simulink model "Test2_1"  (R2021a)
(part 2 of 2)

  Line 89 : spsDistributedParametersLineLib/Distributed Parameters Line  Phases=3  Length=0.02  Frequency=50  Resistance=[0.646656091154803 0.0486237908083191 0.0486712220507153;0.0486237908083191 0.646561225344642 0.0486237934466192;0.0486712220507153 0.0486237934466192 0.646656091154803]  Inductance=[0.00282448912315926 0.00133270803418135 0.00132951476746136;0.00133270803418135 0.00282479813276775 0.00133799988507366;0.00132951476746136 0.00133799988507366 0.00282448912315926]  Capacitance=[7.89543174552926e-09 -1.85986777702161e-09 -1.7901190036642e-09;-1.85986777702161e-09 7.82540023894543e-09 -1.8957321828871e-09;-1.7901190036642e-09 -1.8957321828871e-09 7.91264394645417e-09]  x1=[153.230370640917 2391.26534326387 2395.45779665592;314.159265358979 314.159265358979 314.159265358979;0.9381426054202 -0.865117419435394 -2.43426019857906]  x2=[153.230402844459 2391.26073889825 2395.45319480697;314.159265358979 314.159265358979 314.159265358979;0.93814254539382 -0.865117633756149 -2.43426040689413]  x3=[0.134091150426205 5.82873242831537 5.88568625716513;314.159265358979 314.159265358979 314.159265358979;0.931522107244716 -0.837575635614275 -2.40695052925784]  x4=[0.133861464896509 6.3462381763928 6.40423326646663;314.159265358979 314.159265358979 314.159265358979;0.944744271874414 -0.890435947392576 -2.45938130511451]  x5=9.5829454252223e-08  V1=ones(3,3)  V2=ones(3,3)  I1=ones(3,3)  I2=ones(3,3)  nHarmo=1  Measurements=None  Decoupling=off  VsMag0=0  VrMag0=0  VsAngle0=0  VrAngle0=0  IsMag0=0  IrMag0=0  IsAngle0=0  IrAngle0=0
      settings: SourceProductBaseCode=PS
  Line 9 : spsDistributedParametersLineLib/Distributed Parameters Line  Phases=3  Length=0.02  Frequency=50  Resistance=[0.646656091154803 0.0486237908083191 0.0486712220507153;0.0486237908083191 0.646561225344642 0.0486237934466192;0.0486712220507153 0.0486237934466192 0.646656091154803]  Inductance=[0.00282448912315926 0.00133270803418135 0.00132951476746136;0.00133270803418135 0.00282479813276775 0.00133799988507366;0.00132951476746136 0.00133799988507366 0.00282448912315926]  Capacitance=[7.89543174552926e-09 -1.85986777702161e-09 -1.7901190036642e-09;-1.85986777702161e-09 7.82540023894543e-09 -1.8957321828871e-09;-1.7901190036642e-09 -1.8957321828871e-09 7.91264394645417e-09]  x1=[139.613784628439 4217.52722308047 4217.62642474081;314.159265358979 314.159265358979 314.159265358979;0.931225166408948 1.89080004922946 -2.8202976922573]  x2=[139.613822815392 4217.52006491205 4217.61927834542;314.159265358979 314.159265358979 314.159265358979;0.931225429888519 1.89079965963336 -2.82029807495107]  x3=[0.123373305824632 10.2981496913263 10.380801790438;314.159265358979 314.159265358979 314.159265358979;0.926779421621701 1.91078292702978 -2.8004554345958]  x4=[0.120765224807825 11.1715858882522 11.2542853331702;314.159265358979 314.159265358979 314.159265358979;0.935736759138729 1.87235633522372 -2.83862312372742]  x5=9.5829454252223e-08  V1=ones(3,3)  V2=ones(3,3)  I1=ones(3,3)  I2=ones(3,3)  nHarmo=1  Measurements=None  Decoupling=off  VsMag0=0  VrMag0=0  VsAngle0=0  VrAngle0=0  IsMag0=0  IrMag0=0  IsAngle0=0  IrAngle0=0
      settings: SourceProductBaseCode=PS
  Line im1 : spsDistributedParametersLineLib/Distributed Parameters Line  Phases=3  Length=1e-10  Frequency=50  Resistance=[0.646656091154803 0.0486237908083191 0.0486712220507153;0.0486237908083191 0.646561225344642 0.0486237934466192;0.0486712220507153 0.0486237934466192 0.646656091154803]  Inductance=[0.00282448912315926 0.00133270803418135 0.00132951476746136;0.00133270803418135 0.00282479813276775 0.00133799988507366;0.00132951476746136 0.00133799988507366 0.00282448912315926]  Capacitance=[7.89543174552926e-09 -1.85986777702161e-09 -1.7901190036642e-09;-1.85986777702161e-09 7.82540023894543e-09 -1.8957321828871e-09;-1.7901190036642e-09 -1.8957321828871e-09 7.91264394645417e-09]  x1=[139.600491467614 4218.81584590389 4218.91451607394;314.159265358979 314.159265358979 314.159265358979;0.93120240765686 1.89102757934652 -2.82007159456862]  x2=[139.600491467484 4218.81584590393 4218.91451607418;314.159265358979 314.159265358979 314.159265358979;0.931202407653615 1.89102757934648 -2.82007159456862]  x3=[2.39495104418877 10.0531520558199 13.4523376279678;314.159265358979 314.159265358979 314.159265358979;-2.07306138977406 1.7159728748214 -2.96321720619588]  x4=[2.63858020709018 11.6972228256435 8.53725478011855;314.159265358979 314.159265358979 314.159265358979;1.05327657505423 2.04091940379862 -2.59297720135789]  x5=4.79147271261115e-16  V1=ones(3,3)  V2=ones(3,3)  I1=ones(3,3)  I2=ones(3,3)  nHarmo=1  Measurements=None  Decoupling=off  VsMag0=0  VrMag0=0  VsAngle0=0  VrAngle0=0  IsMag0=0  IrMag0=0  IsAngle0=0  IrAngle0=0
      settings: SourceProductBaseCode=PS
  Line im2 : spsDistributedParametersLineLib/Distributed Parameters Line  Phases=3  Length=1e-10  Frequency=50  Resistance=[0.646656091154803 0.0486237908083191 0.0486712220507153;0.0486237908083191 0.646561225344642 0.0486237934466192;0.0486712220507153 0.0486237934466192 0.646656091154803]  Inductance=[0.00282448912315926 0.00133270803418135 0.00132951476746136;0.00133270803418135 0.00282479813276775 0.00133799988507366;0.00132951476746136 0.00133799988507366 0.00282448912315926]  Capacitance=[7.89543174552926e-09 -1.85986777702161e-09 -1.7901190036642e-09;-1.85986777702161e-09 7.82540023894543e-09 -1.8957321828871e-09;-1.7901190036642e-09 -1.8957321828871e-09 7.91264394645417e-09]  x1=[153.212558124086 2392.15576627611 2396.34818431222;314.159265358979 314.159265358979 314.159265358979;0.938198757168088 -0.864957859131465 -2.4341019124231]  x2=[153.212558124091 2392.15576627603 2396.34818431214;314.159265358979 314.159265358979 314.159265358979;0.938198757168096 -0.864957859131481 -2.43410191242311]  x3=[0.150374507197116 4.9941389131791 5.06923933643373;314.159265358979 314.159265358979 314.159265358979;0.783798645997587 -0.817862247865617 -2.376387681184]  x4=[0.120456415579041 7.18402866882818 7.23580636001522;314.159265358979 314.159265358979 314.159265358979;1.11210397866224 -0.897495860417821 -2.47460068555332]  x5=4.79147271261115e-16  V1=ones(3,3)  V2=ones(3,3)  I1=ones(3,3)  I2=ones(3,3)  nHarmo=1  Measurements=None  Decoupling=off  VsMag0=0  VrMag0=0  VsAngle0=0  VrAngle0=0  IsMag0=0  IrMag0=0  IsAngle0=0  IrAngle0=0
      settings: SourceProductBaseCode=PS
  Line im3 : spsDistributedParametersLineLib/Distributed Parameters Line  Phases=3  Length=1e-10  Frequency=50  Resistance=[0.646656091154803 0.0486237908083191 0.0486712220507153;0.0486237908083191 0.646561225344642 0.0486237934466192;0.0486712220507153 0.0486237934466192 0.646656091154803]  Inductance=[0.00282448912315926 0.00133270803418135 0.00132951476746136;0.00133270803418135 0.00282479813276775 0.00133799988507366;0.00132951476746136 0.00133799988507366 0.00282448912315926]  Capacitance=[7.89543174552926e-09 -1.85986777702161e-09 -1.7901190036642e-09;-1.85986777702161e-09 7.82540023894543e-09 -1.8957321828871e-09;-1.7901190036642e-09 -1.8957321828871e-09 7.91264394645417e-09]  x1=[138.811982406861 4221.87237170443 4226.20282418839;314.159265358979 314.159265358979 314.159265358979;0.909247916230907 -0.556815898274562 -2.12771519143661]  x2=[138.811982407814 4221.8723715327 4226.20282401679;314.159265358979 314.159265358979 314.159265358979;0.909247916234134 -0.556815898289708 -2.12771519145178]  x3=[5.7114352671611 2399.57047495897 2405.23950831528;314.159265358979 314.159265358979 314.159265358979;0.198532164333906 2.27374576995704 0.707186662876006]  x4=[5.52541559624089 2420.03219700396 2425.91155689626;314.159265358979 314.159265358979 314.159265358979;-2.97166603107008 -0.865128065419886 -2.43170878274322]  x5=4.79147271261115e-16  V1=ones(3,3)  V2=ones(3,3)  I1=ones(3,3)  I2=ones(3,3)  nHarmo=1  Measurements=None  Decoupling=off  VsMag0=0  VrMag0=0  VsAngle0=0  VrAngle0=0  IsMag0=0  IrMag0=0  IsAngle0=0  IrAngle0=0
      settings: SourceProductBaseCode=PS
  Load {1..2,11,13,8041,8173} (6 alike) : spsThreePhaseSeriesRLCLoadLib/Three-Phase Series RLC Load  LConnTagsString=A|B|C  Configuration=Delta  NominalVoltage=11000  Vabc=[1e3 1e3 1e3]  Vabcp=[1e3 1e3 1e3]  NominalFrequency=50  UnbalancedPower=off  ActivePower=28052.64  InductivePower=13586.514  CapacitivePower=0  Pabc=[10e3 9e3 11e3]  QLabc=[100 90 110]  QCabc=[100 90 110]  Pabcp=[10e3 9e3 11e3]  QLabcp=[100 90 110]  QCabcp=[100 90 110]  Measurements=None  LoadType=constant Z
  Load 10 : spsThreePhaseSeriesRLCLoadLib/Three-Phase Series RLC Load  LConnTagsString=A|B|C  Configuration=Delta  NominalVoltage=11000  Vabc=[1e3 1e3 1e3]  Vabcp=[1e3 1e3 1e3]  NominalFrequency=50  UnbalancedPower=off  ActivePower=17532.9  InductivePower=8491.571  CapacitivePower=0  Pabc=[10e3 9e3 11e3]  QLabc=[100 90 110]  QCabc=[100 90 110]  Pabcp=[10e3 9e3 11e3]  QLabcp=[100 90 110]  QCabcp=[100 90 110]  Measurements=None  LoadType=constant Z
  Load 12 : spsThreePhaseSeriesRLCLoadLib/Three-Phase Series RLC Load  LConnTagsString=A|B|C  Configuration=Delta  NominalVoltage=11000  Vabc=[1e3 1e3 1e3]  Vabcp=[1e3 1e3 1e3]  NominalFrequency=50  UnbalancedPower=off  ActivePower=17532.9  InductivePower=8491.571  CapacitivePower=0  Pabc=[10e3 9e3 11e3]  QLabc=[100 90 110]  QCabc=[100 90 110]  Pabcp=[10e3 9e3 11e3]  QLabcp=[100 90 110]  QCabcp=[100 90 110]  Measurements=None  LoadType=constant Z
  Load {3,6,14,17,8287,8485} (6 alike) : spsThreePhaseSeriesRLCLoadLib/Three-Phase Series RLC Load  LConnTagsString=A|B|C  Configuration=Delta  NominalVoltage=11000  Vabc=[1e3 1e3 1e3]  Vabcp=[1e3 1e3 1e3]  NominalFrequency=50  UnbalancedPower=off  ActivePower=35065.8  InductivePower=16983.142  CapacitivePower=0  Pabc=[10e3 9e3 11e3]  QLabc=[100 90 110]  QCabc=[100 90 110]  Pabcp=[10e3 9e3 11e3]  QLabcp=[100 90 110]  QCabcp=[100 90 110]  Measurements=None  LoadType=constant Z
  Load {4,9,15,20,8293,8733} (6 alike) : spsThreePhaseSeriesRLCLoadLib/Three-Phase Series RLC Load  LConnTagsString=A|B|C  Configuration=Delta  NominalVoltage=11000  Vabc=[1e3 1e3 1e3]  Vabcp=[1e3 1e3 1e3]  NominalFrequency=50  UnbalancedPower=off  ActivePower=7013.16  InductivePower=3396.628  CapacitivePower=0  Pabc=[10e3 9e3 11e3]  QLabc=[100 90 110]  QCabc=[100 90 110]  Pabcp=[10e3 9e3 11e3]  QLabcp=[100 90 110]  QCabcp=[100 90 110]  Measurements=None  LoadType=constant Z
  Load {5,7,16,18,8424,8551} (6 alike) : spsThreePhaseSeriesRLCLoadLib/Three-Phase Series RLC Load  LConnTagsString=A|B|C  Configuration=Delta  NominalVoltage=11000  Vabc=[1e3 1e3 1e3]  Vabcp=[1e3 1e3 1e3]  NominalFrequency=50  UnbalancedPower=off  ActivePower=11221.056  InductivePower=5434.605  CapacitivePower=0  Pabc=[10e3 9e3 11e3]  QLabc=[100 90 110]  QCabc=[100 90 110]  Pabcp=[10e3 9e3 11e3]  QLabcp=[100 90 110]  QCabcp=[100 90 110]  Measurements=None  LoadType=constant Z
  Load 19 : spsThreePhaseSeriesRLCLoadLib/Three-Phase Series RLC Load  LConnTagsString=A|B|C  Configuration=Delta  NominalVoltage=11000  Vabc=[1e3 1e3 1e3]  Vabcp=[1e3 1e3 1e3]  NominalFrequency=50  UnbalancedPower=off  ActivePower=280.526  InductivePower=135.865  CapacitivePower=0  Pabc=[10e3 9e3 11e3]  QLabc=[100 90 110]  QCabc=[100 90 110]  Pabcp=[10e3 9e3 11e3]  QLabcp=[100 90 110]  QCabcp=[100 90 110]  Measurements=None  LoadType=constant Z
  Load 8 : spsThreePhaseSeriesRLCLoadLib/Three-Phase Series RLC Load  LConnTagsString=A|B|C  Configuration=Delta  NominalVoltage=11000  Vabc=[1e3 1e3 1e3]  Vabcp=[1e3 1e3 1e3]  NominalFrequency=50  UnbalancedPower=off  ActivePower=280.526  InductivePower=135.865  CapacitivePower=0  Pabc=[10e3 9e3 11e3]  QLabc=[100 90 110]  QCabc=[100 90 110]  Pabcp=[10e3 9e3 11e3]  QLabcp=[100 90 110]  QCabcp=[100 90 110]  Measurements=None  LoadType=constant Z
  Load 8605 : spsThreePhaseSeriesRLCLoadLib/Three-Phase Series RLC Load  LConnTagsString=A|B|C  Configuration=Delta  NominalVoltage=11000  Vabc=[1e3 1e3 1e3]  Vabcp=[1e3 1e3 1e3]  NominalFrequency=50  UnbalancedPower=off  ActivePower=280.526  InductivePower=135.865  CapacitivePower=0  Pabc=[10e3 9e3 11e3]  QLabc=[100 90 110]  QCabc=[100 90 110]  Pabcp=[10e3 9e3 11e3]  QLabcp=[100 90 110]  QCabcp=[100 90 110]  Measurements=None  LoadType=constant Z
  Load 8737 : spsThreePhaseSeriesRLCLoadLib/Three-Phase Series RLC Load  LConnTagsString=A|B|C  Configuration=Delta  NominalVoltage=11000  Vabc=[1e3 1e3 1e3]  Vabcp=[1e3 1e3 1e3]  NominalFrequency=50  UnbalancedPower=off  ActivePower=17532.9  InductivePower=8491.571  CapacitivePower=0  Pabc=[10e3 9e3 11e3]  QLabc=[100 90 110]  QCabc=[100 90 110]  Pabcp=[10e3 9e3 11e3]  QLabcp=[100 90 110]  QCabcp=[100 90 110]  Measurements=None  LoadType=constant Z
  R{1..3,5} (4 alike) : spsThreePhaseVIMeasurementLib/Three-Phase V-I Measurement  VoltageMeasurement=phase-to-ground  SetLabelV=off  LabelV=Vabc  Vpu=off  VpuLL=off  CurrentMeasurement=yes  SetLabelI=off  LabelI=Iabc  Ipu=off  Pbase=100e6  Vbase=500e3  OutputType=Complex  PhasorSimulation=on  PSBequivalent=0
  Scope R{1..3,5} (4 alike) : Scope  NumInputPorts=2
  Source PC1_TT2 : spsThreePhaseSourceLib/Three-Phase Source  InternalConnection=Yn  VoltagePhases=off  Voltage=10000  PhaseAngle=0  Voltage_phases=[25e3 25e3 25e3]/sqrt(3)  PhaseAngles_phases=[0 -120 +120]  Frequency=50  NonIdealSource=on  SpecifyImpedance=off  Resistance=0.14  Inductance=0.0031831  ShortCircuitLevel=100e6  BaseVoltage=25e3  XRratio=7  BusType=swing  Pref=10e3  Qref=0  Prefabc=[10e3, 10e3, 10e3]  Qrefabc=[0, 0, 0]  Qmin=-inf  Qmax=inf
  Source Zn : spsSeriesRLCBranchLib/Series RLC Branch  LConnTagsString=__new0  RConnTagsString=__new0  BranchType=RL  Resistance=0.001  Inductance=3.1831e-06  SetiL0=off  InitialCurrent=0  Capacitance=0  Setx0=off  InitialVoltage=0  Measurements=None
  powergui : spspowerguiLib/powergui  Priority=1  SimulationMode=Phasor  SampleTime=50e-6  frequency=50  Iterations=50  frequencyindice=50  Pbase=100e6  ErrMax=1e-4  UnitsV=kV  UnitsW=MW  buscounter=0  FunctionMessages=off  echomessages=off  EnableUseOfTLC=off  CurrentSourceSwitches=off  DisableSnubberDevices=off  DisableRonSwitches=off  DisableVfSwitches=off  DisplayEquations=off  AutomaticDiscreteSolvers=off  SolverType=Tustin/Backward Euler (TBE)  Interpol=off  ExternalGateDelay=off  methode=off  Ts=10  x0status=blocks  SPID=off  SwTol=0  HookPort=off  NonlinearTolerance=1e-4  nMaxIteration=100  ContinueOnMaxIteration=off  RestoreLinks=warning  ResistiveCurrentMeasurement=off  Frange=[0:2:500]  Ylog=off  Xlog=on  ShowGrid=off  save=off  variable=ZData  structure=0  ZoomFFT=off  StartTime=0.0  cycles=1  DisplayStyle=1  fundamental=60  FreqAxis=off  MaxFrequency=1000  frequencyindicesteady=1  RmsSteady=1  display=off
  wires:
  R5/1 -> Scope R5/1
  R2/2 -> Scope R2/2
  R2/1 -> Scope R2/1
  R5/2 -> Scope R5/2
  R1/2 -> Scope R1/2
  R1/1 -> Scope R1/1
  R3/2 -> Scope R3/2
  R3/1 -> Scope R3/1
  connections:
  Source Zn/RConn1 -- Source PC1_TT2/LConn1
  Source Zn/LConn1 -- Ground/LConn1
  Line 58/LConn1 -- Line 57/LConn1 -- Line 56/RConn1
  Line 58/LConn2 -- Line 57/LConn2 -- Line 56/RConn2
  Line 58/LConn3 -- Line 57/LConn3 -- Line 56/RConn3
  Line 81/RConn1 -- Load 11/LConn1
  Line 81/RConn2 -- Load 11/LConn2
  Line 81/RConn3 -- Load 11/LConn3
  Load 20/LConn1 -- Line 42/RConn1
  Load 20/LConn2 -- Line 42/RConn2
  Load 20/LConn3 -- Line 42/RConn3
  Line 49/LConn1 -- Line 48/LConn1 -- Line 47/RConn1
  Line 49/LConn2 -- Line 48/LConn2 -- Line 47/RConn2
  Line 49/LConn3 -- Line 48/LConn3 -- Line 47/RConn3
  Line 28/RConn1 -- Load 1/LConn1
  Line 28/RConn2 -- Load 1/LConn2
  Line 28/RConn3 -- Load 1/LConn3
  Line 23/RConn1 -- Load 8/LConn1
  Line 23/RConn2 -- Load 8/LConn2
  Line 23/RConn3 -- Load 8/LConn3
  Line 74/LConn1 -- R2/RConn1
  Line 74/LConn2 -- R2/RConn2
  Line 74/LConn3 -- R2/RConn3
  Line 15/LConn1 -- Line 14/LConn1 -- Line 13/RConn1
  Line 15/LConn2 -- Line 14/LConn2 -- Line 13/RConn2
  Line 15/LConn3 -- Line 14/LConn3 -- Line 13/RConn3
  Line 17/LConn1 -- Line 16/LConn1 -- Line im1/RConn1
  Line 17/LConn2 -- Line 16/LConn2 -- Line im1/RConn2
  Line 16/LConn3 -- Line 17/LConn3 -- Line im1/RConn3
  Line 20/LConn1 -- Line 19/LConn1 -- Line 21/RConn1
  Line 20/LConn2 -- Line 19/LConn2 -- Line 21/RConn2
  Line 20/LConn3 -- Line 19/LConn3 -- Line 21/RConn3
  Load 13/LConn1 -- Line 83/LConn1 -- Line 87/RConn1 -- Line 41/LConn1
  Load 13/LConn2 -- Line 83/LConn2 -- Line 87/RConn2 -- Line 41/LConn2
  Line 41/LConn3 -- Load 13/LConn3 -- Line 87/RConn3 -- Line 83/LConn3
  Line im2/LConn1 -- R3/RConn1
  Line im2/LConn2 -- R3/RConn2
  Line im2/LConn3 -- R3/RConn3
  Line 19/RConn1 -- R1/LConn1
  Line 19/RConn2 -- R1/LConn2
  Line 19/RConn3 -- R1/LConn3
  Load 10/LConn1 -- Line 9/RConn1
  Load 10/LConn2 -- Line 9/RConn2
  Load 10/LConn3 -- Line 9/RConn3
  Source PC1_TT2/RConn1 -- R2/LConn1
  Source PC1_TT2/RConn2 -- R2/LConn2
  Source PC1_TT2/RConn3 -- R2/LConn3
  Line 71/LConn1 -- Line 70/LConn1 -- Line 72/RConn1
  Line 71/LConn2 -- Line 70/LConn2 -- Line 72/RConn2
  Line 71/LConn3 -- Line 70/LConn3 -- Line 72/RConn3
  Load 6/LConn1 -- Line 21/LConn1 -- Line 22/RConn1
  Load 6/LConn2 -- Line 21/LConn2 -- Line 22/RConn2
  Load 6/LConn3 -- Line 21/LConn3 -- Line 22/RConn3
  Line 23/LConn1 -- Line 22/LConn1 -- Line 24/RConn1
  Line 23/LConn2 -- Line 22/LConn2 -- Line 24/RConn2
  Line 23/LConn3 -- Line 22/LConn3 -- Line 24/RConn3
  Line 37/LConn1 -- Line 38/LConn1 -- Line im2/RConn1
  Line 37/LConn2 -- Line 38/LConn2 -- Line im2/RConn2
  Line 37/LConn3 -- Line 38/LConn3 -- Line im2/RConn3
  Load 8173/LConn1 -- Line 50/RConn1 -- Line 45/LConn1 -- Line 46/LConn1
  Load 8173/LConn2 -- Line 50/RConn2 -- Line 45/LConn2 -- Line 46/LConn2
  Load 8173/LConn3 -- Line 50/RConn3 -- Line 45/LConn3 -- Line 46/LConn3
  Line 66/RConn1 -- Load 8605/LConn1
  Line 66/RConn2 -- Load 8605/LConn2
  Line 66/RConn3 -- Load 8605/LConn3
  Load 17/LConn1 -- Line 43/LConn1 -- Line 75/RConn1
  Load 17/LConn2 -- Line 43/LConn2 -- Line 75/RConn2
  Load 17/LConn3 -- Line 43/LConn3 -- Line 75/RConn3
  Line 30/LConn1 -- Line 41/RConn1
  Line 30/LConn2 -- Line 41/RConn2
  Line 30/LConn3 -- Line 41/RConn3
  Line im3/LConn1 -- R5/RConn1
  Line im3/LConn2 -- R5/RConn2
  Line im3/LConn3 -- R5/RConn3
  Load 12/LConn1 -- Line 89/RConn1
  Load 12/LConn2 -- Line 89/RConn2
  Load 12/LConn3 -- Line 89/RConn3
  Line 54/LConn1 -- Line 53/LConn1 -- Line 59/RConn1
  Line 54/LConn2 -- Line 53/LConn2 -- Line 59/RConn2
  Line 54/LConn3 -- Line 53/LConn3 -- Line 59/RConn3
  Line 36/LConn1 -- Line 35/LConn1 -- Line 34/RConn1
  Line 36/LConn2 -- Line 35/LConn2 -- Line 34/RConn2
  Line 36/LConn3 -- Line 35/LConn3 -- Line 34/RConn3
  Line 56/LConn1 -- Line 55/LConn1 -- Line 54/RConn1
  Line 56/LConn2 -- Line 55/LConn2 -- Line 54/RConn2
  Line 56/LConn3 -- Line 55/LConn3 -- Line 54/RConn3
  Line 58/RConn1 -- Load 8551/LConn1
  Line 58/RConn2 -- Load 8551/LConn2
  Line 58/RConn3 -- Load 8551/LConn3
  Line 33/RConn1 -- Load 16/LConn1
  Line 33/RConn2 -- Load 16/LConn2
  Line 33/RConn3 -- Load 16/LConn3
  Line 14/RConn1 -- Load 4/LConn1
  Line 14/RConn2 -- Load 4/LConn2
  Line 14/RConn3 -- Load 4/LConn3
  Line 60/LConn1 -- Line 59/LConn1 -- Line im3/RConn1
  Line 60/LConn2 -- Line 59/LConn2 -- Line im3/RConn2
  Line 60/LConn3 -- Line 59/LConn3 -- Line im3/RConn3
  Line 71/RConn1 -- Load 8041/LConn1
  Line 71/RConn2 -- Load 8041/LConn2
  Line 71/RConn3 -- Load 8041/LConn3
  Line 73/LConn1 -- Line 74/RConn1
  Line 73/LConn2 -- Line 74/RConn2
  Line 73/LConn3 -- Line 74/RConn3
  Line 46/RConn1 -- Line 47/LConn1
  Line 46/RConn2 -- Line 47/LConn2
  Line 46/RConn3 -- Line 47/LConn3
  Line 36/RConn1 -- Load 18/LConn1
  Line 36/RConn2 -- Load 18/LConn2
  Line 36/RConn3 -- Load 18/LConn3
  Line 60/RConn1 -- Line 61/LConn1
  Line 60/RConn2 -- Line 61/LConn2
  Line 60/RConn3 -- Line 61/LConn3
  Line 38/RConn1 -- Line 39/LConn1
  Line 38/RConn2 -- Line 39/LConn2
  Line 38/RConn3 -- Line 39/LConn3
  Load 9/LConn1 -- Line 20/RConn1
  Load 9/LConn2 -- Line 20/RConn2
  Load 9/LConn3 -- Line 20/RConn3
  Line 26/RConn1 -- Load 3/LConn1
  Line 26/RConn2 -- Load 3/LConn2
  Line 26/RConn3 -- Load 3/LConn3
  Load 8485/LConn1 -- Line 64/LConn1 -- Line 65/RConn1
  Load 8485/LConn2 -- Line 64/LConn2 -- Line 65/RConn2
  Load 8485/LConn3 -- Line 64/LConn3 -- Line 65/RConn3
  Line 31/LConn1 -- Line 32/LConn1 -- Line 37/RConn1
  Line 32/LConn2 -- Line 31/LConn2 -- Line 37/RConn2
  Line 32/LConn3 -- Line 31/LConn3 -- Line 37/RConn3
  Line 89/LConn1 -- Line 88/LConn1 -- Line 31/RConn1
  Line 88/LConn2 -- Line 89/LConn2 -- Line 31/RConn2
  Line 89/LConn3 -- Line 88/LConn3 -- Line 31/RConn3
  Line 3/RConn1 -- Line 4/LConn1
  Line 3/RConn2 -- Line 4/LConn2
  Line 3/RConn3 -- Line 4/LConn3
  Line 15/RConn1 -- Load 7/LConn1
  Line 15/RConn2 -- Load 7/LConn2
  Line 15/RConn3 -- Load 7/LConn3
  Line 72/LConn1 -- Line 73/RConn1
  Line 72/LConn2 -- Line 73/RConn2
  Line 72/LConn3 -- Line 73/RConn3
  Line 25/LConn1 -- Line 24/LConn1 -- Line 27/RConn1
  Line 25/LConn2 -- Line 24/LConn2 -- Line 27/RConn2
  Line 25/LConn3 -- Line 24/LConn3 -- Line 27/RConn3
  Line 40/RConn1 -- R3/LConn1
  Line 40/RConn2 -- R3/LConn2
  Line 40/RConn3 -- R3/LConn3
  Line 8/LConn1 -- Line 9/LConn1 -- Line 10/RConn1
  Line 8/LConn2 -- Line 9/LConn2 -- Line 10/RConn2
  Line 8/LConn3 -- Line 9/LConn3 -- Line 10/RConn3
  Line 49/RConn1 -- Line 82/LConn1
  Line 49/RConn2 -- Line 82/LConn2
  Line 49/RConn3 -- Line 82/LConn3
  Line 17/RConn1 -- Line 18/LConn1
  Line 17/RConn2 -- Line 18/LConn2
  Line 17/RConn3 -- Line 18/LConn3
  Load 8737/LConn1 -- Line 52/RConn1
  Load 8737/LConn2 -- Line 52/RConn2
  Load 8737/LConn3 -- Line 52/RConn3
  Line 13/LConn1 -- Line 12/LConn1 -- Line 11/RConn1
  Line 13/LConn2 -- Line 12/LConn2 -- Line 11/RConn2
  Line 13/LConn3 -- Line 12/LConn3 -- Line 11/RConn3
  Load 8733/LConn1 -- Line 63/RConn1
  Load 8733/LConn2 -- Line 63/RConn2
  Load 8733/LConn3 -- Line 63/RConn3
  Line 42/LConn1 -- Line 40/LConn1 -- Line 43/RConn1
  Line 42/LConn2 -- Line 40/LConn2 -- Line 43/RConn2
  Line 42/LConn3 -- Line 40/LConn3 -- Line 43/RConn3
  Line 68/LConn1 -- Line 67/LConn1 -- Line 70/RConn1
  Line 68/LConn2 -- Line 67/LConn2 -- Line 70/RConn2
  Line 68/LConn3 -- Line 67/LConn3 -- Line 70/RConn3
  Line 76/LConn1 -- Line 75/LConn1 -- Line 77/RConn1
  Line 76/LConn2 -- Line 75/LConn2 -- Line 77/RConn2
  Line 76/LConn3 -- Line 75/LConn3 -- Line 77/RConn3
  Line 1/LConn1 -- Line 2/RConn1
  Line 1/LConn2 -- Line 2/RConn2
  Line 1/LConn3 -- Line 2/RConn3
  Line 68/RConn1 -- Line 69/LConn1
  Line 68/RConn2 -- Line 69/LConn2
  Line 68/RConn3 -- Line 69/LConn3
  Line 55/RConn1 -- Load 8424/LConn1
  Line 55/RConn2 -- Load 8424/LConn2
  Line 55/RConn3 -- Load 8424/LConn3
  Line 6/LConn1 -- Line 5/LConn1 -- Line 4/RConn1
  Line 6/LConn2 -- Line 5/LConn2 -- Line 4/RConn2
  Line 6/LConn3 -- Line 5/LConn3 -- Line 4/RConn3
  Line 8/RConn1 -- Line 7/LConn1
  Line 8/RConn2 -- Line 7/LConn2
  Line 8/RConn3 -- Line 7/LConn3
  Line 69/RConn1 -- Load 8287/LConn1
  Line 69/RConn2 -- Load 8287/LConn2
  Line 69/RConn3 -- Load 8287/LConn3
  Line 63/LConn1 -- Line 62/LConn1 -- Line 64/RConn1
  Line 63/LConn2 -- Line 62/LConn2 -- Line 64/RConn2
  Line 63/LConn3 -- Line 62/LConn3 -- Line 64/RConn3
  Line 57/RConn1 -- Load 8293/LConn1
  Line 57/RConn2 -- Load 8293/LConn2
  Line 57/RConn3 -- Load 8293/LConn3
  Line 34/LConn1 -- Line 33/LConn1 -- Line 32/RConn1
  Line 34/LConn2 -- Line 33/LConn2 -- Line 32/RConn2
  Line 34/LConn3 -- Line 33/LConn3 -- Line 32/RConn3
  Line 83/RConn1 -- Line 84/LConn1
  Line 83/RConn2 -- Line 84/LConn2
  Line 83/RConn3 -- Line 84/LConn3
  Line 51/RConn1 -- Line 50/LConn1
  Line 51/RConn2 -- Line 50/LConn2
  Line 51/RConn3 -- Line 50/LConn3
  Line 78/RConn1 -- Line 79/LConn1
  Line 78/RConn2 -- Line 79/LConn2
  Line 78/RConn3 -- Line 79/LConn3
  Line 86/LConn1 -- Line 85/LConn1 -- Line 84/RConn1
  Line 86/LConn2 -- Line 85/LConn2 -- Line 84/RConn2
  Line 85/LConn3 -- Line 86/LConn3 -- Line 84/RConn3
  Line 88/RConn1 -- Line 87/LConn1
  Line 88/RConn2 -- Line 87/LConn2
  Line 88/RConn3 -- Line 87/LConn3
  Line 66/LConn1 -- Line 65/LConn1 -- Line 67/RConn1
  Line 66/LConn2 -- Line 65/LConn2 -- Line 67/RConn2
  Line 66/LConn3 -- Line 65/LConn3 -- Line 67/RConn3
  Line 62/RConn1 -- R5/LConn1
  Line 62/RConn2 -- R5/LConn2
  Line 62/RConn3 -- R5/LConn3
  Load 2/LConn1 -- Line 7/RConn1 -- Line 3/LConn1 -- Line 2/LConn1
  Load 2/LConn2 -- Line 7/RConn2 -- Line 3/LConn2 -- Line 2/LConn2
  Load 2/LConn3 -- Line 7/RConn3 -- Line 3/LConn3 -- Line 2/LConn3
  Line im1/LConn1 -- R1/RConn1
  Line im1/LConn2 -- R1/RConn2
  Line im1/LConn3 -- R1/RConn3
  Line 76/RConn1 -- Load 19/LConn1
  Line 76/RConn2 -- Load 19/LConn2
  Line 76/RConn3 -- Load 19/LConn3
  Line 11/LConn1 -- Line 10/LConn1 -- Line 16/RConn1
  Line 11/LConn2 -- Line 10/LConn2 -- Line 16/RConn2
  Line 11/LConn3 -- Line 10/LConn3 -- Line 16/RConn3
  Line 28/LConn1 -- Line 27/LConn1 -- Line 29/RConn1
  Line 28/LConn2 -- Line 27/LConn2 -- Line 29/RConn2
  Line 28/LConn3 -- Line 27/LConn3 -- Line 29/RConn3
  Line 35/RConn1 -- Load 15/LConn1
  Line 35/RConn2 -- Load 15/LConn2
  Line 35/RConn3 -- Load 15/LConn3
  Line 61/RConn1 -- Line 29/LConn3
  Line 61/RConn2 -- Line 29/LConn2
  Line 61/RConn3 -- Line 29/LConn1
  Line 81/LConn1 -- Line 80/LConn1 -- Line 82/RConn1
  Line 81/LConn2 -- Line 80/LConn2 -- Line 82/RConn2
  Line 81/LConn3 -- Line 80/LConn3 -- Line 82/RConn3
  Line 78/LConn1 -- Line 77/LConn1 -- Line 80/RConn1
  Line 78/LConn2 -- Line 77/LConn2 -- Line 80/RConn2
  Line 78/LConn3 -- Line 77/LConn3 -- Line 80/RConn3
  Line 25/RConn1 -- Line 26/LConn1
  Line 25/RConn2 -- Line 26/LConn2
  Line 25/RConn3 -- Line 26/LConn3
  Line 12/RConn1 -- Load 5/LConn1
  Line 12/RConn2 -- Load 5/LConn2
  Line 12/RConn3 -- Load 5/LConn3
  Line 79/RConn1 -- Load 14/LConn1
  Line 79/RConn2 -- Load 14/LConn2
  Line 79/RConn3 -- Load 14/LConn3
  Line 44/LConn1 -- Line 45/RConn1
  Line 44/LConn2 -- Line 45/RConn2
  Line 44/LConn3 -- Line 45/RConn3
  Line 51/LConn1 -- Line 52/LConn1 -- Line 53/RConn1
  Line 51/LConn2 -- Line 52/LConn2 -- Line 53/RConn2
  Line 51/LConn3 -- Line 52/LConn3 -- Line 53/RConn3
